simulink model "Automatic_Transmission"  (R2020b)
settings: Solver=VariableStepAuto  StartTime=0.0  StopTime=10.0  RelTol=1e-3
values from neighbouring files (symbols this model uses):
  Iei = 0.0219914882836    [Automatic_Transmission_data.mat]
undefined symbols (not defined in the file or in its folder): Rfd, Rw, sigbuilder_block, v
settings Model: Creator=Shivashis  LastModifiedBy=Shivashis

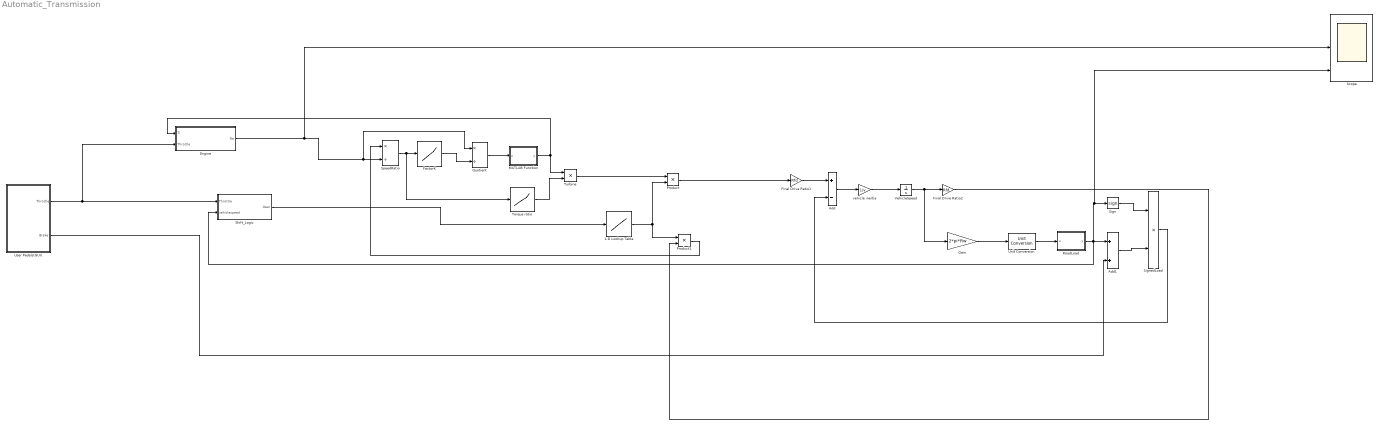
== system Automatic_Transmission ==
  1-D Lookup Table : Lookup_n-D  NumberOfTableDimensions=1  BreakpointsForDimension1=[-5:5]  Table=tanh([-5:5])  InternalRulePriority=Speed  RndMeth=Simplest  InputSameDT=on
  Add : Sum  Inputs=+-
  Add1 : Sum
  Engine : Subsystem
  FactorK : Lookup_n-D  NumberOfTableDimensions=1  BreakpointsForDimension1=[-5:5]  Table=tanh([-5:5])  InternalRulePriority=Speed  RndMeth=Simplest  InputSameDT=on
  Final Drive Ratio1 : Gain  Gain=Rfd
  Final Drive Ratio2 : Gain  Gain=Rfd
  Gain : Gain  Gain=2*pi*Rw
  MATLAB Function : MATLAB Function  TreatAsAtomicUnit=on
  Product : Product
  Product1 : Product
  Quotient : Product  Inputs=*/
  RoadLoad : MATLAB Function  TreatAsAtomicUnit=on
  Scope : Scope  NumInputPorts=3
  Shift_Logic : Stateflow chart  TreatAsAtomicUnit=on
  Sign : Signum
  SignedLoad : Product
  SpeedRatio : Product  Inputs=*/
  Torque ratio : Lookup_n-D  NumberOfTableDimensions=1  BreakpointsForDimension1=[-5:5]  Table=tanh([-5:5])  InternalRulePriority=Speed  RndMeth=Simplest  InputSameDT=on
  Turbine : Product
  Unit Conversion : UnitConversion
  User Pedals(GUI) : Subsystem  Tag=STV Subsys  LoadFcn=sigbuilder_block('load');  StartFcn=sigbuilder_block('start');  StopFcn=sigbuilder_block('stop');  ClipboardFcn=sigbuilder_block('clipboard');  mask(Sigbuilder block){tuvar=[0:10]}
      mask help: Simulink:masks:SigbuilderBlock_MD
      mask init:
      | if ~strcmp(get_param(bdroot(gcbh),'SimulationStatus'),'stopped') tuvar = sigbuilder_block('maskInit'); end
      settings: CopyFcn=sigbuilder_block('copy');  DeleteFcn=sigbuilder_block('delete');  ModelCloseFcn=sigbuilder_block('modelClose');  PreSaveFcn=sigbuilder_block('preSave');  PauseFcn=sigbuilder_block('pause');  ContinueFcn=sigbuilder_block('continue');  NameChangeFcn=sigbuilder_block('namechange');  OpenFcn=sigbuilder_block('open',[6 30 1012.5 447.75 ]);  CloseFcn=sigbuilder_block('close');
      mask Display: plot(0, 0, 100, 100,[2, 2, 32, 32, 2], [68, 8, 8, 68, 68],[32, 2], [38, 38], [32, 19, 2],[53, 60, 44], [32, 17, 17, 2],[16, 16, 31, 31]);txt = getActiveGroup(gcbh);text(2, 100, txt,'verticalAlignment', 'top');
  VehicleSpeed : Integrator
  vehicle inertia : Gain  Gain=1/v
  wires:
  SpeedRatio/1 -> Torque ratio/1, FactorK/1
  FactorK/1 -> Quotient/2
  Quotient/1 -> MATLAB Function/1(u)
  MATLAB Function/1(y) -> Engine/1(Ti), Turbine/1
  Torque ratio/1 -> Turbine/2
  Turbine/1 -> Product/1
  Shift_Logic/1(Gear) -> 1-D Lookup Table/1
  1-D Lookup Table/1 -> Product/2, Product1/1
  Product/1 -> Final Drive Ratio1/1
  Final Drive Ratio1/1 -> Add/1
  Add/1 -> vehicle inertia/1
  vehicle inertia/1 -> VehicleSpeed/1
  VehicleSpeed/1 -> Gain/1, Final Drive Ratio2/1
  Gain/1 -> Unit Conversion/1
  Unit Conversion/1 -> RoadLoad/1(u)
  Add1/1 -> SignedLoad/2
  Sign/1 -> SignedLoad/1
  RoadLoad/1(y) -> Scope/3, Sign/1, Shift_Logic/2(vehiclespeed), Add1/1
  SignedLoad/1 -> Add/2
  Product1/1 -> SpeedRatio/1
  User Pedals(GUI)/1(Throttle) -> Engine/2(Throttle), Shift_Logic/1(Throttle)
  User Pedals(GUI)/2(Brake) -> Add1/2
  Final Drive Ratio2/1 -> Product1/2
  Engine/1(Ne) -> Scope/2, Quotient/1, SpeedRatio/2

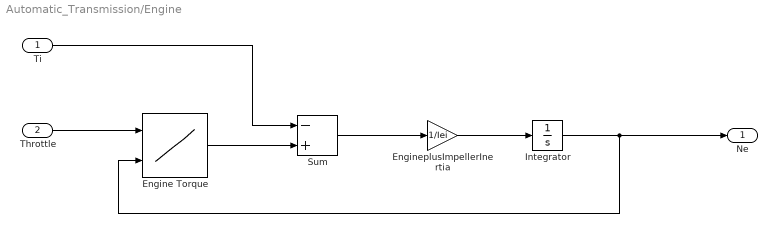
== system Automatic_Transmission/Engine ==
  Ti : Inport
  Throttle : Inport  Port=2
  Engine Torque : Lookup_n-D  BreakpointsForDimension1=[1:3]  BreakpointsForDimension2=[1:3]  InternalRulePriority=Speed  RndMeth=Simplest  InputSameDT=on
      settings: InputPortMap=u0,u1
  EngineplusImpellerInertia : Gain  Gain=1/Iei
  Integrator : Integrator
  Sum : Sum  Inputs=-+
  Ne : Outport
  wires:
  Throttle/1 -> Engine Torque/1
  Sum/1 -> EngineplusImpellerInertia/1
  Engine Torque/1 -> Sum/2
  EngineplusImpellerInertia/1 -> Integrator/1
  Ti/1 -> Sum/1
  Integrator/1 -> Engine Torque/2, Ne/1

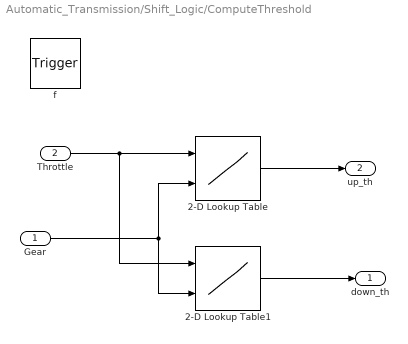
== system Automatic_Transmission/Shift_Logic/ComputeThreshold ==
  Gear : Inport  OutDataTypeStr=double  PortDimensions=1
  Throttle : Inport  Port=2  OutDataTypeStr=double  PortDimensions=1
  f : TriggerPort  TriggerType=function-call  VariantControl=(inherit)
      settings: CopyFcn=Stateflow.SLINSF.SimulinkMan.removeBlockPreDeleteFcn  PreDeleteFcn=Stateflow.SLINSF.SimulinkMan.unsafePredeleteFcn
  2-D Lookup Table : Lookup_n-D  BreakpointsForDimension1=[1:3]  BreakpointsForDimension2=[1:3]  InternalRulePriority=Speed  RndMeth=Simplest  InputSameDT=on
      settings: InputPortMap=u0,u1
  2-D Lookup Table1 : Lookup_n-D  BreakpointsForDimension1=[1:3]  BreakpointsForDimension2=[1:3]  InternalRulePriority=Speed  RndMeth=Simplest  InputSameDT=on
      settings: InputPortMap=u0,u1
  down_th : Outport
  up_th : Outport  Port=2
  wires:
  Throttle/1 -> 2-D Lookup Table1/1, 2-D Lookup Table/1
  2-D Lookup Table/1 -> up_th/1
  2-D Lookup Table1/1 -> down_th/1
  Gear/1 -> 2-D Lookup Table/2, 2-D Lookup Table1/2

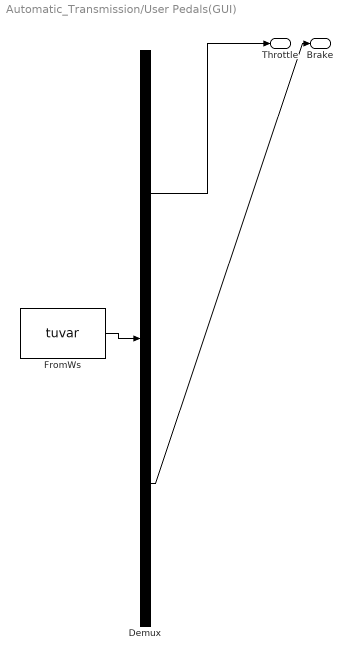
== system Automatic_Transmission/User Pedals(GUI) ==
  Demux : Demux  Tag=STV Demux  Outputs=2
      settings: DisplayOption=none
  FromWs : FromWorkspace  Tag=STV FromWs  VariableName=tuvar
      SigBuilderData=|
      | common.afterFinalStr = 'Extrapolate'
      | common.sampleTime = 0
      | dataSet.timeRange = [0 50]
      | dataSet.name = 'Group 1'
      | sbobj.Groups.Name = 'Group 1'
      | sbobj.Groups.Signals(1).Name = 'Throttle'
      | sbobj.Groups.Signals(1).XData = [0 15 15 50]
      | sbobj.Groups.Signals(1).YData = [60 40 101 60]
      | sbobj.Groups.Signals(2).Name = 'Brake'
      | sbobj.Groups.Signals(2).XData = [0 50]
      | sbobj.Groups.Signals(2).YData = [0 0]
      | sbobj.Groups.TimeRange = [0 50]
  Throttle : Outport  Tag=STV Outport
  Brake : Outport  Tag=STV Outport  Port=2
  wires:
  FromWs/1 -> Demux/1
  Demux/1 -> Throttle/1
  Demux/2 -> Brake/1

== matlab function Automatic_Transmission/RoadLoad ==
  data: u input; y output
function y = fcn(u)

y = rload0 + rload2*u^2;

== matlab function Automatic_Transmission/MATLAB Function ==
  data: u input; y output
function y = fcn(u)

y = u^2;

== stateflow chart Automatic_Transmission/Shift_Logic ==
  state Gear_state [parallel]
    settings: executionOrder=1
    state First
      entry:
      Gear=1;
    state Second
      entry:
      Gear=2;
    state Third
      entry:
      Gear=3;
    state Fourth
      entry:
      Gear=4;
    (default) -> First
    Third -> Fourth [order 1] : UP
    Second -> Third [order 1] : UP
    First -> Second : UP
    Fourth -> Third : DOWN
    Third -> Second [order 2] : DOWN
    Second -> First [order 2] : DOWN
  state Selection_state [parallel]
    during:
    [down_th,up_th]=ComputeThreshold(Gear,Throttle);
    settings: executionOrder=2
    state Steady_state
    state Downshifting
    state Upshifting
    (default) -> Steady_state
    Steady_state -> Downshifting [order 2] : [vehiclespeed<down_th]
    Steady_state -> Upshifting [order 1] : [vehiclespeed>up_th]
    Downshifting -> Steady_state [order 1] : after(TWAIT,tick)
        | [vehiclespeed<=down_th]
        | {Gear_state.DOWN}
    Downshifting -> Steady_state [order 2] : [vehiclespeed>down_th]
    Upshifting -> Steady_state [order 1] : after(TWAIT,tick)
        | [vehiclespeed>=up_th]
        | {Gear_state.UP}
    Upshifting -> Steady_state [order 2] : [vehiclespeed<up_th]
  state [down_th,up_th]=ComputeThreshold(Gear,Throttle) [function]
  data: Gear function_input double size=1; Throttle function_input double size=1; down_th function_output; up_th function_output; Throttle input double; Gear output fixdt(0,8,5); vehiclespeed input fixdt(0,8,5)
